simulink model "Demo002ADAS"  (Simulink 8.3)
settings: Solver=ode45  StartTime=0.0  StopTime=10.0  RelTol=1e-3
model workspace (MAT data in the model file):
  MPS_Models = {'..\..\..\solutions\demos\models\demos\Demo002.mps'}
  variantInfo = VariabilitySupport
  variantInfo.name = 'ADASVariabilityModel'
  variantInfo.configModels = VariantConfigurationModel
  variantInfo.configModels.id = '4psHK0ldtYh'
  variantInfo.configModels.name = 'PL_OEM1_AB01'
  variantInfo.configModels.featureRef = MpsObjectRef
  variantInfo.configModels.featureRef.targetNodeId = '4psHK0ldtYc'
  variantInfo.configModels.featureRef.resolveInfo = 'ADASVariabilityMdl'
  variantInfo.configModels.rootFeature = VariantSelectedFeature
  variantInfo.configModels.rootFeature.featureRef = MpsObjectRef
  variantInfo.configModels.rootFeature.featureRef.targetNodeId = '4psHK0ldtYd'
  variantInfo.configModels.rootFeature.featureRef.resolveInfo = 'ADASVariabilityMdl_root'
  variantInfo.configModels.rootFeature.children(1) = VariantSelectedFeature
  variantInfo.configModels.rootFeature.children(1).featureRef = MpsObjectRef
  variantInfo.configModels.rootFeature.children(1).featureRef.targetNodeId = '2wirY2bY5pP'
  variantInfo.configModels.rootFeature.children(1).featureRef.resolveInfo = 'ProductLine'
  variantInfo.configModels.rootFeature.children(1).children(1) = VariantSelectedFeature
  variantInfo.configModels.rootFeature.children(1).children(1).featureRef = MpsObjectRef
  variantInfo.configModels.rootFeature.children(1).children(1).featureRef.targetNodeId = '63tTPuP4CV9'
  variantInfo.configModels.rootFeature.children(1).children(1).featureRef.resolveInfo = 'Sensors'
  variantInfo.configModels.rootFeature.children(1).children(1).children = VariantSelectedFeature
  variantInfo.configModels.rootFeature.children(1).children(1).children.featureRef = MpsObjectRef
  variantInfo.configModels.rootFeature.children(1).children(1).children.featureRef.targetNodeId = '6jJ$2DnCoYq'
  variantInfo.configModels.rootFeature.children(1).children(1).children.featureRef.resolveInfo = 'Camera'
  variantInfo.configModels.rootFeature.children(1).children(1).children.children = VariantSelectedFeature
  variantInfo.configModels.rootFeature.children(1).children(1).children.children.featureRef = MpsObjectRef
  variantInfo.configModels.rootFeature.children(1).children(1).children.children.featureRef.targetNodeId = '6jJ$2DnCptI'
  variantInfo.configModels.rootFeature.children(1).children(1).children.children.featureRef.resolveInfo = 'C1'
  variantInfo.configModels.rootFeature.children(1).children(2) = VariantSelectedFeature
  variantInfo.configModels.rootFeature.children(1).children(2).featureRef = MpsObjectRef
  variantInfo.configModels.rootFeature.children(1).children(2).featureRef.targetNodeId = '6jJ$2DnCqGP'
  variantInfo.configModels.rootFeature.children(1).children(2).featureRef.resolveInfo = 'Actuators'
  variantInfo.configModels.rootFeature.children(1).children(2).children(1) = VariantSelectedFeature
  variantInfo.configModels.rootFeature.children(1).children(2).children(1).featureRef = MpsObjectRef
  variantInfo.configModels.rootFeature.children(1).children(2).children(1).featureRef.targetNodeId = '6jJ$2DnCqHv'
  variantInfo.configModels.rootFeature.children(1).children(2).children(1).featureRef.resolveInfo = 'PT'
  variantInfo.configModels.rootFeature.children(1).children(2).children(1).children = VariantSelectedFeature
  variantInfo.configModels.rootFeature.children(1).children(2).children(1).children.featureRef = MpsObjectRef
  variantInfo.configModels.rootFeature.children(1).children(2).children(1).children.featureRef.targetNodeId = '6jJ$2DnCqIu'
  variantInfo.configModels.rootFeature.children(1).children(2).children(1).children.featureRef.resolveInfo = 'G1'
  variantInfo.configModels.rootFeature.children(1).children(2).children(2) = VariantSelectedFeature
  variantInfo.configModels.rootFeature.children(1).children(2).children(2).featureRef = MpsObjectRef
  variantInfo.configModels.rootFeature.children(1).children(2).children(2).featureRef.targetNodeId = '6jJ$2DnCqHy'
  variantInfo.configModels.rootFeature.children(1).children(2).children(2).featureRef.resolveInfo = 'Brakes'
  variantInfo.configModels.rootFeature.children(1).children(2).children(2).children = VariantSelectedFeature
  variantInfo.configModels.rootFeature.children(1).children(2).children(2).children.featureRef = MpsObjectRef
  variantInfo.configModels.rootFeature.children(1).children(2).children(2).children.featureRef.targetNodeId = '6jJ$2DnCqYd'
  variantInfo.configModels.rootFeature.children(1).children(2).children(2).children.featureRef.resolveInfo = 'H1'
  variantInfo.configModels.rootFeature.children(1).children(2).children(3) = VariantSelectedFeature
  variantInfo.configModels.rootFeature.children(1).children(2).children(3).featureRef = MpsObjectRef
  variantInfo.configModels.rootFeature.children(1).children(2).children(3).featureRef.targetNodeId = '6jJ$2DnCqH_'
  variantInfo.configModels.rootFeature.children(1).children(2).children(3).featureRef.resolveInfo = 'Steering'
  variantInfo.configModels.rootFeature.children(1).children(2).children(3).children = VariantSelectedFeature
  variantInfo.configModels.rootFeature.children(1).children(2).children(3).children.featureRef = MpsObjectRef
  variantInfo.configModels.rootFeature.children(1).children(2).children(3).children.featureRef.targetNodeId = '6jJ$2DnCrdZ'
  variantInfo.configModels.rootFeature.children(1).children(2).children(3).children.featureRef.resolveInfo = 'I1'
  variantInfo.configModels.rootFeature.children(1).children(2).children(4) = VariantSelectedFeature
  variantInfo.configModels.rootFeature.children(1).children(2).children(4).featureRef = MpsObjectRef
  variantInfo.configModels.rootFeature.children(1).children(2).children(4).featureRef.targetNodeId = '6jJ$2DnCqHD'
  variantInfo.configModels.rootFeature.children(1).children(2).children(4).featureRef.resolveInfo = 'Headlight'
  variantInfo.configModels.rootFeature.children(1).children(2).children(4).children = VariantSelectedFeature
  variantInfo.configModels.rootFeature.children(1).children(2).children(4).children.featureRef = MpsObjectRef
  variantInfo.configModels.rootFeature.children(1).children(2).children(4).children.featureRef.targetNodeId = '6jJ$2DnCJBB'
  variantInfo.configModels.rootFeature.children(1).children(2).children(4).children.featureRef.resolveInfo = 'ToHLComm'
  variantInfo.configModels.rootFeature.children(1).children(2).children(5) = VariantSelectedFeature
  variantInfo.configModels.rootFeature.children(1).children(2).children(5).featureRef = MpsObjectRef
  variantInfo.configModels.rootFeature.children(1).children(2).children(5).featureRef.targetNodeId = '6jJ$2DnCqHI'
  variantInfo.configModels.rootFeature.children(1).children(2).children(5).featureRef.resolveInfo = 'IP'
  variantInfo.configModels.rootFeature.children(1).children(2).children(5).children = VariantSelectedFeature
  variantInfo.configModels.rootFeature.children(1).children(2).children(5).children.featureRef = MpsObjectRef
  variantInfo.configModels.rootFeature.children(1).children(2).children(5).children.featureRef.targetNodeId = '6jJ$2DnCrHG'
  variantInfo.configModels.rootFeature.children(1).children(2).children(5).children.featureRef.resolveInfo = 'K1'
  variantInfo.configModels.rootFeature.children(1).children(3) = VariantSelectedFeature
  variantInfo.configModels.rootFeature.children(1).children(3).featureRef = MpsObjectRef
  variantInfo.configModels.rootFeature.children(1).children(3).featureRef.targetNodeId = '63tTPuP4CVo'
  variantInfo.configModels.rootFeature.children(1).children(3).featureRef.resolveInfo = 'region'
  variantInfo.configModels.rootFeature.children(1).children(3).children = VariantSelectedFeature
  variantInfo.configModels.rootFeature.children(1).children(3).children.featureRef = MpsObjectRef
  variantInfo.configModels.rootFeature.children(1).children(3).children.featureRef.targetNodeId = '63tTPuP4CVv'
  variantInfo.configModels.rootFeature.children(1).children(3).children.featureRef.resolveInfo = 'Germany'
  variantInfo.configModels.rootFeature.children(1).children(4) = VariantSelectedFeature
  variantInfo.configModels.rootFeature.children(1).children(4).featureRef = MpsObjectRef
  variantInfo.configModels.rootFeature.children(1).children(4).featureRef.targetNodeId = '6jJ$2DnCrX_'
  variantInfo.configModels.rootFeature.children(1).children(4).featureRef.resolveInfo = 'MajorFunctions'
  variantInfo.configModels.rootFeature.children(1).children(4).children = VariantSelectedFeature
  variantInfo.configModels.rootFeature.children(1).children(4).children.featureRef = MpsObjectRef
  variantInfo.configModels.rootFeature.children(1).children(4).children.featureRef.targetNodeId = '6jJ$2DnCrYD'
  variantInfo.configModels.rootFeature.children(1).children(4).children.featureRef.resolveInfo = 'TSR'
  variantInfo.configModels.rootFeature.children(1).children(5) = VariantSelectedFeature
  variantInfo.configModels.rootFeature.children(1).children(5).featureRef = MpsObjectRef
  variantInfo.configModels.rootFeature.children(1).children(5).featureRef.targetNodeId = '6jJ$2DnCJfc'
  variantInfo.configModels.rootFeature.children(1).children(5).featureRef.resolveInfo = 'Customer'
  variantInfo.configModels.rootFeature.children(1).children(6) = VariantSelectedFeature
  variantInfo.configModels.rootFeature.children(1).children(6).featureRef = MpsObjectRef
  variantInfo.configModels.rootFeature.children(1).children(6).featureRef.targetNodeId = '6jJ$2DnCJd5'
  variantInfo.configModels.rootFeature.children(1).children(6).featureRef.resolveInfo = 'Comm'
  variantInfo.configModels.rootFeature.children(2) = VariantSelectedFeature
  variantInfo.configModels.rootFeature.children(2).featureRef = MpsObjectRef
  variantInfo.configModels.rootFeature.children(2).featureRef.targetNodeId = '2wirY2bYc6v'
  variantInfo.configModels.rootFeature.children(2).featureRef.resolveInfo = 'ProductTesting'
  variantInfo.configModels.rootFeature.children(2).children = VariantSelectedFeature
  variantInfo.configModels.rootFeature.children(2).children.featureRef = MpsObjectRef
  variantInfo.configModels.rootFeature.children(2).children.featureRef.targetNodeId = '2wirY2bYc8b'
  variantInfo.configModels.rootFeature.children(2).children.featureRef.resolveInfo = 'MIL'
PreLoadFcn:
  | VarScript002ADAS
PostLoadFcn:
  | loadDRIReqsInfo('Demo002ADAS', []);
PreSaveFcn:
  | modelWS=get_param('Demo002ADAS', 'modelworkspace');modelWS.evalin('clear driModuleInfo simModuleInfo');clear modelWS;
settings Model: Creator=swami  LastModifiedBy=swami
settings DataIOCC: SignalLoggingSaveFormat=Dataset
settings DebuggingCC: UnderspecifiedInitializationDetection=Simplified  StateNameClashWarn=none
settings GRTTargetCC: CombineOutputUpdateFcns=on  GRTInterface=off

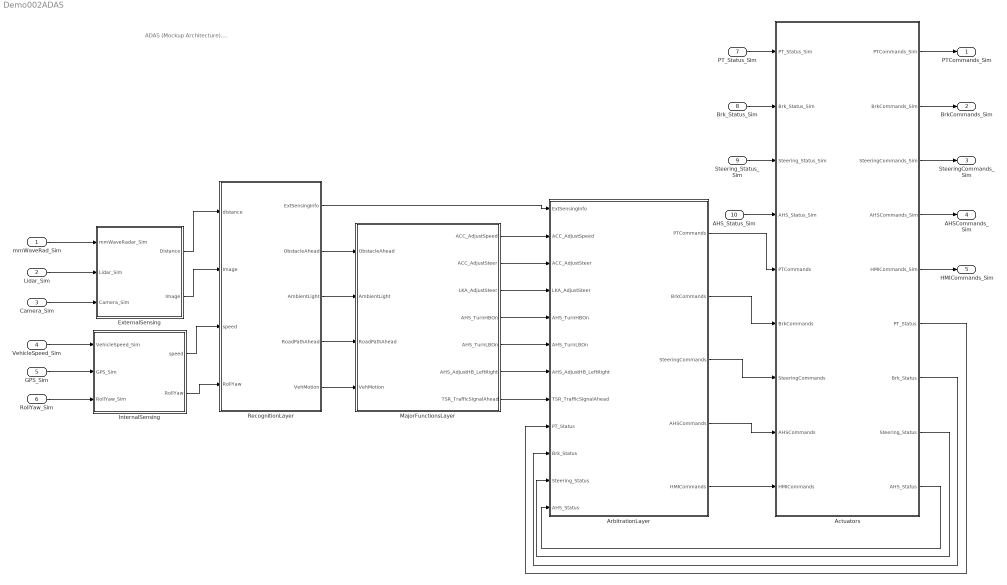
== system Demo002ADAS ==
  note: ADAS (Mockup Architecture)....
  mmWaveRad_Sim : Inport
  Lidar_Sim : Inport  Port=2
  Camera_Sim : Inport  Port=3
  VehicleSpeed_Sim : Inport  Port=4
  GPS_Sim : Inport  Port=5
  RollYaw_Sim : Inport  Port=6
  PT_Status_Sim : Inport  Port=7
  Brk_Status_Sim : Inport  Port=8
  Steering_Status_Sim : Inport  Port=9
  AHS_Status_Sim : Inport  Port=10
  Actuators : Subsystem
  ArbitrationLayer : Subsystem
  ExternalSensing : Subsystem
  InternalSensing : Subsystem
  MajorFunctionsLayer : Subsystem
  RecognitionLayer : Subsystem
  PTCommands_Sim : Outport
  BrkCommands_Sim : Outport  Port=2
  SteeringCommands_Sim : Outport  Port=3
  AHSCommands_Sim : Outport  Port=4
  HMICommands_Sim : Outport  Port=5
  wires:
  MajorFunctionsLayer/1(ACC_AdjustSpeed) -> ArbitrationLayer/2(ACC_AdjustSpeed)
  MajorFunctionsLayer/2(ACC_AdjustSteer) -> ArbitrationLayer/3(ACC_AdjustSteer)
  MajorFunctionsLayer/3(LKA_AdjustSteer) -> ArbitrationLayer/4(LKA_AdjustSteer)
  MajorFunctionsLayer/4(AHS_TurnHBOn) -> ArbitrationLayer/5(AHS_TurnHBOn)
  MajorFunctionsLayer/5(AHS_TurnLBOn) -> ArbitrationLayer/6(AHS_TurnLBOn)
  MajorFunctionsLayer/6(AHS_AdjustHB_LeftRight) -> ArbitrationLayer/7(AHS_AdjustHB_LeftRight)
  MajorFunctionsLayer/7(TSR_TrafficSignalAhead) -> ArbitrationLayer/8(TSR_TrafficSIgnalAhead)
  RecognitionLayer/2(ObstacleAhead) -> MajorFunctionsLayer/1(ObstacleAhead)
  RecognitionLayer/3(AmbientLight) -> MajorFunctionsLayer/2(AmbientLight)
  RecognitionLayer/4(RoadPathAhead) -> MajorFunctionsLayer/3(RoadPathAhead)
  RecognitionLayer/5(VehMotion) -> MajorFunctionsLayer/4(VehMotion)
  ExternalSensing/2(Image) -> RecognitionLayer/2(Image)
  ExternalSensing/1(Distance) -> RecognitionLayer/1(distance)
  InternalSensing/1(speed) -> RecognitionLayer/3(speed)
  InternalSensing/2(RollYaw) -> RecognitionLayer/4(RollYaw)
  ArbitrationLayer/2(BrkCommands) -> Actuators/6(BrkCommands)
  ArbitrationLayer/4(AHSCommands) -> Actuators/8(AHSCommands)
  ArbitrationLayer/5(HMICommands) -> Actuators/9(HMICommands)
  Actuators/9(AHS_Status) -> ArbitrationLayer/12(AHS_Status)
  RecognitionLayer/1(ExtSensingInfo) -> ArbitrationLayer/1(ExtSensingInfo)
  Actuators/1(PTCommands_Sim) -> PTCommands_Sim/1
  Actuators/2(BrkCommands_Sim) -> BrkCommands_Sim/1
  Actuators/3(SteeringCommands_Sim) -> SteeringCommands_Sim/1
  Actuators/4(AHSCommands_Sim) -> AHSCommands_Sim/1
  Actuators/5(HMICommands_Sim) -> HMICommands_Sim/1
  mmWaveRad_Sim/1 -> ExternalSensing/1(mmWaveRadar_Sim)
  Lidar_Sim/1 -> ExternalSensing/2(Lidar_Sim)
  Camera_Sim/1 -> ExternalSensing/3(Camera_Sim)
  VehicleSpeed_Sim/1 -> InternalSensing/1(VehicleSpeed_Sim)
  RollYaw_Sim/1 -> InternalSensing/3(RollYaw_Sim)
  GPS_Sim/1 -> InternalSensing/2(GPS_Sim)
  Actuators/8(Steering_Status) -> ArbitrationLayer/11(Steering_Status)
  Actuators/7(Brk_Status) -> ArbitrationLayer/10(Brk_Status)
  Actuators/6(PT_Status) -> ArbitrationLayer/9(PT_Status)
  PT_Status_Sim/1 -> Actuators/1(PT_Status_Sim)
  Brk_Status_Sim/1 -> Actuators/2(Brk_Status_Sim)
  Steering_Status_Sim/1 -> Actuators/3(Steering_Status_Sim)
  AHS_Status_Sim/1 -> Actuators/4(AHS_Status_Sim)
  ArbitrationLayer/1(PTCommands) -> Actuators/5(PTCommands)
  ArbitrationLayer/3(SteeringCommands) -> Actuators/7(SteeringCommands)

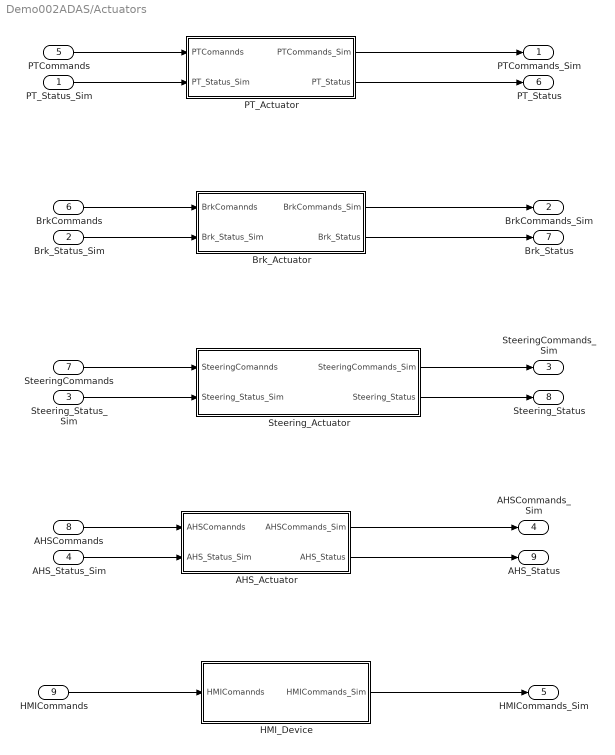
== system Demo002ADAS/Actuators ==
  PT_Status_Sim : Inport
  Brk_Status_Sim : Inport  Port=2
  Steering_Status_Sim : Inport  Port=3
  AHS_Status_Sim : Inport  Port=4
  PTCommands : Inport  Port=5
  BrkCommands : Inport  Port=6
  SteeringCommands : Inport  Port=7
  AHSCommands : Inport  Port=8
  HMICommands : Inport  Port=9
  AHS_Actuator : Subsystem  Variant=on
  Brk_Actuator : Subsystem  Variant=on
  HMI_Device : Subsystem  Variant=on
  PT_Actuator : Subsystem  Variant=on
  Steering_Actuator : Subsystem  Variant=on
  PTCommands_Sim : Outport
  BrkCommands_Sim : Outport  Port=2
  SteeringCommands_Sim : Outport  Port=3
  AHSCommands_Sim : Outport  Port=4
  HMICommands_Sim : Outport  Port=5
  PT_Status : Outport  Port=6
  Brk_Status : Outport  Port=7
  Steering_Status : Outport  Port=8
  AHS_Status : Outport  Port=9
  wires:
  PTCommands/1 -> PT_Actuator/1(PTComannds)
  PT_Actuator/1(PTCommands_Sim) -> PTCommands_Sim/1
  PT_Actuator/2(PT_Status) -> PT_Status/1
  BrkCommands/1 -> Brk_Actuator/1(BrkComannds)
  Brk_Actuator/1(BrkCommands_Sim) -> BrkCommands_Sim/1
  Brk_Actuator/2(Brk_Status) -> Brk_Status/1
  SteeringCommands/1 -> Steering_Actuator/1(SteeringComannds)
  Steering_Actuator/1(SteeringCommands_Sim) -> SteeringCommands_Sim/1
  Steering_Actuator/2(Steering_Status) -> Steering_Status/1
  AHSCommands/1 -> AHS_Actuator/1(AHSComannds)
  AHS_Actuator/1(AHSCommands_Sim) -> AHSCommands_Sim/1
  AHS_Actuator/2(AHS_Status) -> AHS_Status/1
  HMICommands/1 -> HMI_Device/1(HMIComannds)
  HMI_Device/1(HMICommands_Sim) -> HMICommands_Sim/1
  PT_Status_Sim/1 -> PT_Actuator/2(PT_Status_Sim)
  Brk_Status_Sim/1 -> Brk_Actuator/2(Brk_Status_Sim)
  Steering_Status_Sim/1 -> Steering_Actuator/2(Steering_Status_Sim)
  AHS_Status_Sim/1 -> AHS_Actuator/2(AHS_Status_Sim)

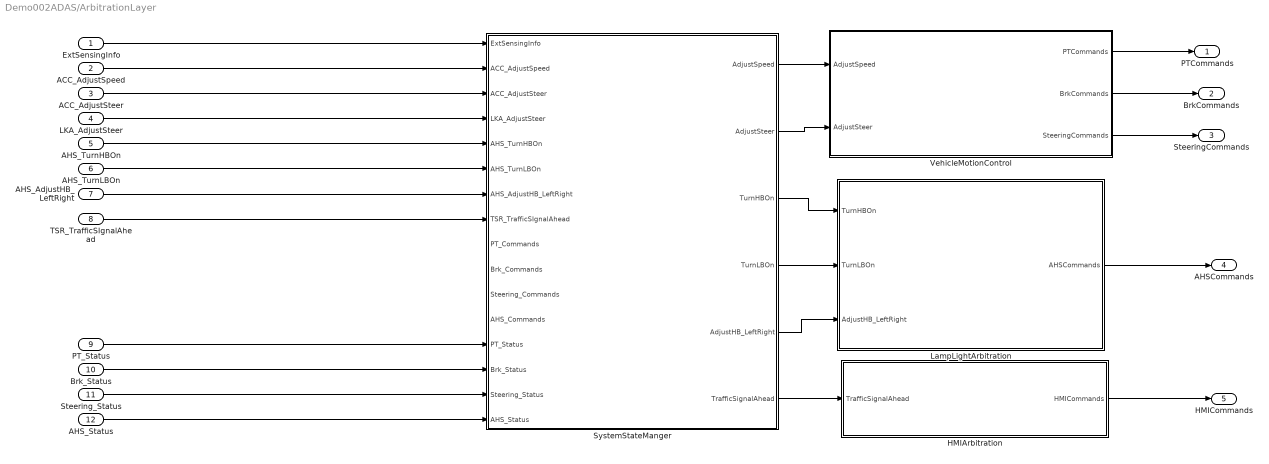
== system Demo002ADAS/ArbitrationLayer ==
  ExtSensingInfo : Inport
  ACC_AdjustSpeed : Inport  Port=2
  ACC_AdjustSteer : Inport  Port=3
  LKA_AdjustSteer : Inport  Port=4
  AHS_TurnHBOn : Inport  Port=5
  AHS_TurnLBOn : Inport  Port=6
  AHS_AdjustHB_LeftRight : Inport  Port=7
  TSR_TrafficSIgnalAhead : Inport  Port=8
  PT_Status : Inport  Port=9
  Brk_Status : Inport  Port=10
  Steering_Status : Inport  Port=11
  AHS_Status : Inport  Port=12
  HMIArbitration : Subsystem  Variant=on
  LampLightArbitration : Subsystem  Variant=on
  SystemStateManger : Subsystem  Variant=on
  VehicleMotionControl : Subsystem
  PTCommands : Outport
  BrkCommands : Outport  Port=2
  SteeringCommands : Outport  Port=3
  AHSCommands : Outport  Port=4
  HMICommands : Outport  Port=5
  wires:
  ACC_AdjustSpeed/1 -> SystemStateManger/2(ACC_AdjustSpeed)
  ACC_AdjustSteer/1 -> SystemStateManger/3(ACC_AdjustSteer)
  LKA_AdjustSteer/1 -> SystemStateManger/4(LKA_AdjustSteer)
  AHS_TurnHBOn/1 -> SystemStateManger/5(AHS_TurnHBOn)
  AHS_TurnLBOn/1 -> SystemStateManger/6(AHS_TurnLBOn)
  AHS_AdjustHB_LeftRight/1 -> SystemStateManger/7(AHS_AdjustHB_LeftRight)
  TSR_TrafficSIgnalAhead/1 -> SystemStateManger/8(TSR_TrafficSIgnalAhead)
  PT_Status/1 -> SystemStateManger/13(PT_Status)
  Brk_Status/1 -> SystemStateManger/14(Brk_Status)
  Steering_Status/1 -> SystemStateManger/15(Steering_Status)
  AHS_Status/1 -> SystemStateManger/16(AHS_Status)
  SystemStateManger/1(AdjustSpeed) -> VehicleMotionControl/1(AdjustSpeed)
  SystemStateManger/2(AdjustSteer) -> VehicleMotionControl/2(AdjustSteer)
  VehicleMotionControl/1(PTCommands) -> PTCommands/1
  VehicleMotionControl/2(BrkCommands) -> BrkCommands/1
  VehicleMotionControl/3(SteeringCommands) -> SteeringCommands/1
  SystemStateManger/3(TurnHBOn) -> LampLightArbitration/1(TurnHBOn)
  SystemStateManger/4(TurnLBOn) -> LampLightArbitration/2(TurnLBOn)
  SystemStateManger/5(AdjustHB_LeftRight) -> LampLightArbitration/3(AdjustHB_LeftRight)
  LampLightArbitration/1(AHSCommands) -> AHSCommands/1
  SystemStateManger/6(TrafficSignalAhead) -> HMIArbitration/1(TrafficSignalAhead)
  HMIArbitration/1(HMICommands) -> HMICommands/1
  ExtSensingInfo/1 -> SystemStateManger/1(ExtSensingInfo)

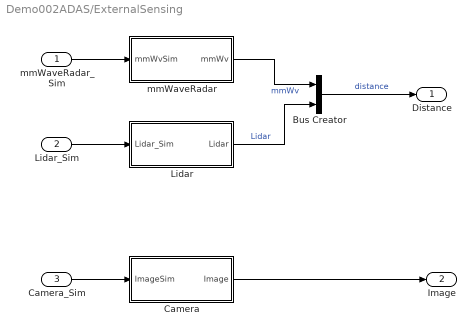
== system Demo002ADAS/ExternalSensing ==
  mmWaveRadar_Sim : Inport
  Lidar_Sim : Inport  Port=2
  Camera_Sim : Inport  Port=3
  Bus Creator : BusCreator  Inputs=2
  Camera : Subsystem  Variant=on
  Lidar : Subsystem  Variant=on
  mmWaveRadar : Subsystem  Variant=on
  Distance : Outport
  Image : Outport  Port=2
  wires:
  mmWaveRadar_Sim/1 -> mmWaveRadar/1(mmWvSim)
  mmWaveRadar/1(mmWv) -> Bus Creator/1  "mmWv"
  Lidar_Sim/1 -> Lidar/1(Lidar_Sim)
  Lidar/1(Lidar) -> Bus Creator/2  "Lidar"
  Bus Creator/1 -> Distance/1  "distance"
  Camera/1(Image) -> Image/1
  Camera_Sim/1 -> Camera/1(ImageSim)

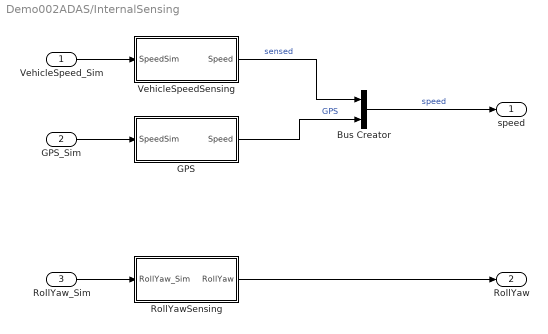
== system Demo002ADAS/InternalSensing ==
  VehicleSpeed_Sim : Inport
  GPS_Sim : Inport  Port=2
  RollYaw_Sim : Inport  Port=3
  Bus Creator : BusCreator  Inputs=2
  GPS : Subsystem  Variant=on
  RollYawSensing : Subsystem  Variant=on
  VehicleSpeedSensing : Subsystem  Variant=on
  speed : Outport
  RollYaw : Outport  Port=2
  wires:
  RollYaw_Sim/1 -> RollYawSensing/1(RollYaw_Sim)
  RollYawSensing/1(RollYaw) -> RollYaw/1
  VehicleSpeed_Sim/1 -> VehicleSpeedSensing/1(SpeedSim)
  GPS_Sim/1 -> GPS/1(SpeedSim)
  VehicleSpeedSensing/1(Speed) -> Bus Creator/1  "sensed"
  GPS/1(Speed) -> Bus Creator/2  "GPS"
  Bus Creator/1 -> speed/1  "speed"

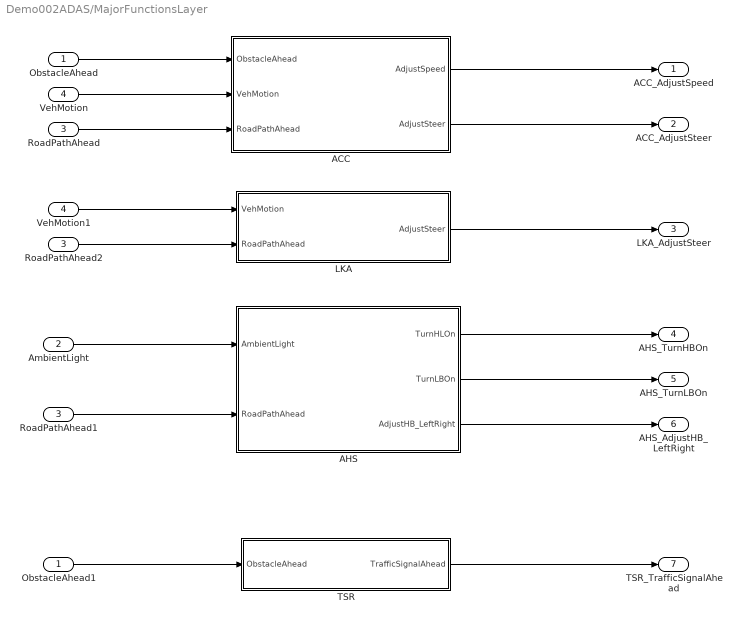
== system Demo002ADAS/MajorFunctionsLayer ==
  ObstacleAhead : Inport
  AmbientLight : Inport  Port=2
  RoadPathAhead : Inport  Port=3
  VehMotion : Inport  Port=4
  ACC : Subsystem  Variant=on
  AHS : Subsystem  Variant=on
  LKA : Subsystem  Variant=on
  ObstacleAhead1 : InportShadow
  RoadPathAhead1 : InportShadow  Port=3
  RoadPathAhead2 : InportShadow  Port=3
  TSR : Subsystem  Variant=on
  VehMotion1 : InportShadow  Port=4
  ACC_AdjustSpeed : Outport
  ACC_AdjustSteer : Outport  Port=2
  LKA_AdjustSteer : Outport  Port=3
  AHS_TurnHBOn : Outport  Port=4
  AHS_TurnLBOn : Outport  Port=5
  AHS_AdjustHB_LeftRight : Outport  Port=6
  TSR_TrafficSignalAhead : Outport  Port=7
  wires:
  LKA/1(AdjustSteer) -> LKA_AdjustSteer/1
  AmbientLight/1 -> AHS/1(AmbientLight)
  TSR/1(TrafficSignalAhead) -> TSR_TrafficSignalAhead/1
  ObstacleAhead/1 -> ACC/1(ObstacleAhead)
  ACC/1(AdjustSpeed) -> ACC_AdjustSpeed/1
  VehMotion1/1 -> LKA/1(VehMotion)
  ObstacleAhead1/1 -> TSR/1(ObstacleAhead)
  ACC/2(AdjustSteer) -> ACC_AdjustSteer/1
  VehMotion/1 -> ACC/2(VehMotion)
  RoadPathAhead/1 -> ACC/3(RoadPathAhead)
  AHS/1(TurnHLOn) -> AHS_TurnHBOn/1
  AHS/2(TurnLBOn) -> AHS_TurnLBOn/1
  AHS/3(AdjustHB_LeftRight) -> AHS_AdjustHB_LeftRight/1
  RoadPathAhead1/1 -> AHS/2(RoadPathAhead)
  RoadPathAhead2/1 -> LKA/2(RoadPathAhead)

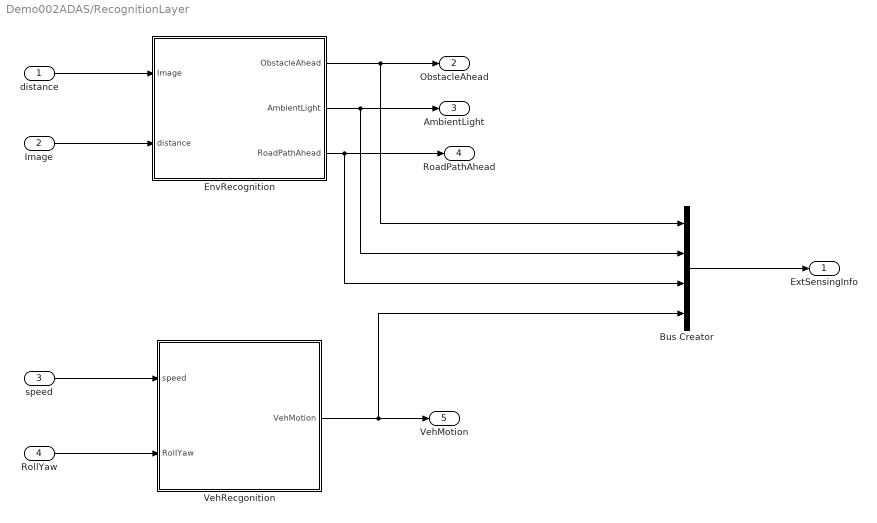
== system Demo002ADAS/RecognitionLayer ==
  distance : Inport
  Image : Inport  Port=2
  speed : Inport  Port=3
  RollYaw : Inport  Port=4
  Bus Creator : BusCreator
  EnvRecognition : Subsystem
  VehRecgonition : Subsystem
  ExtSensingInfo : Outport
  ObstacleAhead : Outport  Port=2
  AmbientLight : Outport  Port=3
  RoadPathAhead : Outport  Port=4
  VehMotion : Outport  Port=5
  wires:
  distance/1 -> EnvRecognition/1(Image)
  Image/1 -> EnvRecognition/2(distance)
  EnvRecognition/1(ObstacleAhead) -> Bus Creator/1, ObstacleAhead/1
  EnvRecognition/2(AmbientLight) -> Bus Creator/2, AmbientLight/1
  speed/1 -> VehRecgonition/1(speed)
  RollYaw/1 -> VehRecgonition/2(RollYaw)
  EnvRecognition/3(RoadPathAhead) -> Bus Creator/3, RoadPathAhead/1
  Bus Creator/1 -> ExtSensingInfo/1
  VehRecgonition/1(VehMotion) -> Bus Creator/4, VehMotion/1

== system Demo002ADAS/Actuators/AHS_Actuator ==
  note: 1) Only subsystems can be added as variant choices at this level
      | 2) Blocks cannot be connected at this level as connectivity is
      | automatically determined at simulation, based on the active variant
  AHSComannds : Inport
  AHS_Status_Sim : Inport  Port=2
  Actuator_J1 : Subsystem  VariantControl=D2_Act_AHS_Actuator_Actuator_J1
  Actuator_J2 : Subsystem  VariantControl=D2_Act_AHS_Actuator_Actuator_J2
  ToHIL : Subsystem  VariantControl=D2_Act_AHS_Actuator_ToHIL
  ToSimulation : Subsystem  VariantControl=D2_Act_AHS_Actuator_ToSimulation
  AHSCommands_Sim : Outport
  AHS_Status : Outport  Port=2

== system Demo002ADAS/Actuators/Brk_Actuator ==
  note: 1) Only subsystems can be added as variant choices at this level
      | 2) Blocks cannot be connected at this level as connectivity is
      | automatically determined at simulation, based on the active variant
  BrkComannds : Inport
  Brk_Status_Sim : Inport  Port=2
  Actuator_H1 : Subsystem  VariantControl=D2_Act_Brk_Actuator_Actuator_H1
  Actuator_H2 : Subsystem  VariantControl=D2_Act_Brk_Actuator_Actuator_H2
  ToHIL : Subsystem  VariantControl=D2_Act_Brk_Actuator_ToHIL
  ToSimulation : Subsystem  VariantControl=D2_Act_Brk_Actuator_ToSimulation
  BrkCommands_Sim : Outport
  Brk_Status : Outport  Port=2

== system Demo002ADAS/Actuators/HMI_Device ==
  note: 1) Only subsystems can be added as variant choices at this level
      | 2) Blocks cannot be connected at this level as connectivity is
      | automatically determined at simulation, based on the active variant
  HMIComannds : Inport
  IP_K1 : Subsystem  VariantControl=D2_Act_HMI_Device_IP_K1
  IP_K2 : Subsystem  VariantControl=D2_Act_HMI_Device_IP_K2
  ToHIL : Subsystem  VariantControl=D2_Act_HMI_Device_ToHIL
  ToSimulation : Subsystem  VariantControl=D2_Act_HMI_Device_ToSimulation
  HMICommands_Sim : Outport

== system Demo002ADAS/Actuators/PT_Actuator ==
  note: 1) Only subsystems can be added as variant choices at this level
      | 2) Blocks cannot be connected at this level as connectivity is
      | automatically determined at simulation, based on the active variant
  PTComannds : Inport
  PT_Status_Sim : Inport  Port=2
  Actuator_G1 : Subsystem  VariantControl=D2_Act_PT_Actuator_Actuator_G1
  Actuator_G2 : Subsystem  VariantControl=D2_Act_PT_Actuator_Actuator_G2
  ToHIL : Subsystem  VariantControl=D2_Act_PT_Actuator_ToHIL
  ToSimulation : Subsystem  VariantControl=D2_Act_PT_Actuator_ToSimulation
  PTCommands_Sim : Outport
  PT_Status : Outport  Port=2

== system Demo002ADAS/Actuators/Steering_Actuator ==
  note: 1) Only subsystems can be added as variant choices at this level
      | 2) Blocks cannot be connected at this level as connectivity is
      | automatically determined at simulation, based on the active variant
  SteeringComannds : Inport
  Steering_Status_Sim : Inport  Port=2
  Actuator_I1 : Subsystem  VariantControl=D2_Act_Steering_Actuator_Actuator_I1
  ToHIL : Subsystem  VariantControl=D2_Act_Steering_Actuator_ToHIL
  ToSimulation : Subsystem  VariantControl=D2_Act_Steering_Actuator_ToSimulation
  SteeringCommands_Sim : Outport
  Steering_Status : Outport  Port=2

== system Demo002ADAS/ArbitrationLayer/HMIArbitration ==
  note: 1) Only subsystems can be added as variant choices at this level
      | 2) Blocks cannot be connected at this level as connectivity is
      | automatically determined at simulation, based on the active variant
  TrafficSignalAhead : Inport
  IP_K1 : Subsystem  VariantControl=D2_AL_HMIArbitration_IP_K1
  IP_K2 : Subsystem  VariantControl=D2_AL_HMIArbitration_IP_K2
  ToSimulationAndHIL : Subsystem  VariantControl=D2_AL_HMIArbitration_ToSimulationAndHIL
  HMICommands : Outport

== system Demo002ADAS/ArbitrationLayer/LampLightArbitration ==
  note: 1) Only subsystems can be added as variant choices at this level
      | 2) Blocks cannot be connected at this level as connectivity is
      | automatically determined at simulation, based on the active variant
  TurnHBOn : Inport
  TurnLBOn : Inport  Port=2
  AdjustHB_LeftRight : Inport  Port=3
  Actuator_J2 : Subsystem  VariantControl=D2_AL_LampLightArbitration_Actuator_J2
  "ToSimulation, HIL, and Actuator_J1" : Subsystem  VariantControl=D2_AL_LampLightArbitration_ToSimulation_HIL_and_Actuator_J1
  AHSCommands : Outport

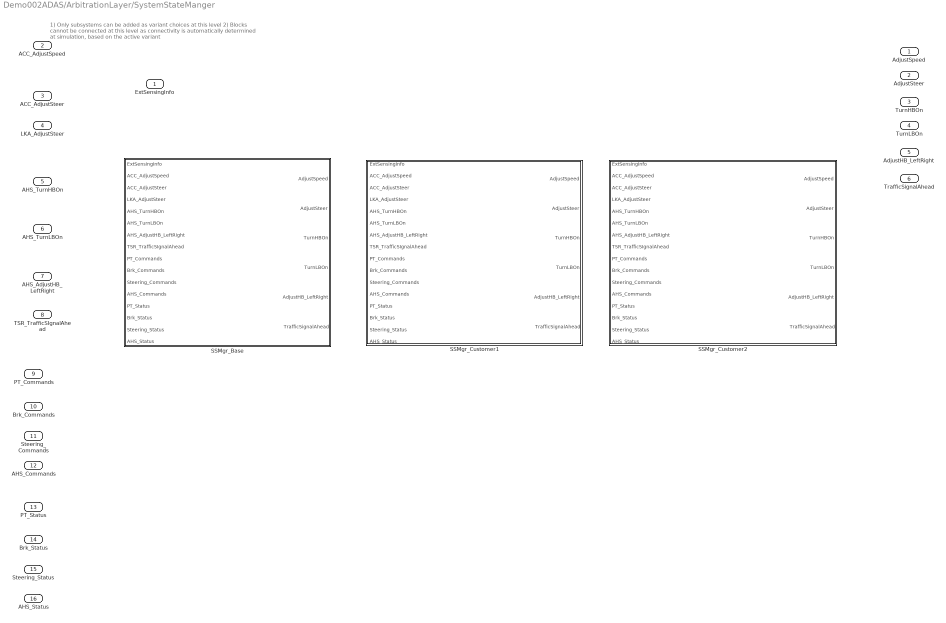
== system Demo002ADAS/ArbitrationLayer/SystemStateManger ==
  note: 1) Only subsystems can be added as variant choices at this level
      | 2) Blocks cannot be connected at this level as connectivity is
      | automatically determined at simulation, based on the active variant
  ExtSensingInfo : Inport
  ACC_AdjustSpeed : Inport  Port=2
  ACC_AdjustSteer : Inport  Port=3
  LKA_AdjustSteer : Inport  Port=4
  AHS_TurnHBOn : Inport  Port=5
  AHS_TurnLBOn : Inport  Port=6
  AHS_AdjustHB_LeftRight : Inport  Port=7
  TSR_TrafficSIgnalAhead : Inport  Port=8
  PT_Commands : Inport  Port=9
  Brk_Commands : Inport  Port=10
  Steering_Commands : Inport  Port=11
  AHS_Commands : Inport  Port=12
  PT_Status : Inport  Port=13
  Brk_Status : Inport  Port=14
  Steering_Status : Inport  Port=15
  AHS_Status : Inport  Port=16
  SSMgr_Base : Subsystem  VariantControl=D2_AL_SystemStateManger_SSMgr_Base
  SSMgr_Customer1 : Subsystem  VariantControl=D2_AL_SystemStateManger_SSMgr_Customer1
  SSMgr_Customer2 : Subsystem  VariantControl=D2_AL_SystemStateManger_SSMgr_Customer2
  AdjustSpeed : Outport
  AdjustSteer : Outport  Port=2
  TurnHBOn : Outport  Port=3
  TurnLBOn : Outport  Port=4
  AdjustHB_LeftRight : Outport  Port=5
  TrafficSignalAhead : Outport  Port=6

== system Demo002ADAS/ArbitrationLayer/VehicleMotionControl ==
  AdjustSpeed : Inport
  AdjustSteer : Inport  Port=2
  ForeAftMotion : Subsystem  Variant=on
  LeftRightMotion : Subsystem  Variant=on
  PTCommands : Outport
  BrkCommands : Outport  Port=2
  SteeringCommands : Outport  Port=3
  wires:
  AdjustSteer/1 -> LeftRightMotion/1(AdjustSteer)
  LeftRightMotion/1(SteeringCommands) -> SteeringCommands/1
  AdjustSpeed/1 -> ForeAftMotion/1(AdjustSpeed)
  ForeAftMotion/1(PTCommands) -> PTCommands/1
  ForeAftMotion/2(BrkCommands) -> BrkCommands/1

== system Demo002ADAS/ExternalSensing/Camera ==
  note: 1) Only subsystems can be added as variant choices at this level
      | 2) Blocks cannot be connected at this level as connectivity is
      | automatically determined at simulation, based on the active variant
  ImageSim : Inport
  FromHIL : Subsystem  VariantControl=D2_XSen_Camera_FromHIL
  FromSimulation : Subsystem  VariantControl=D2_XSen_Camera_FromSimulation
  Sensor_C1 : Subsystem  VariantControl=D2_XSen_Camera_Sensor_C1
  Sensor_C2 : Subsystem  VariantControl=D2_XSen_Camera_Sensor_C2
  Image : Outport

== system Demo002ADAS/ExternalSensing/Lidar ==
  note: 1) Only subsystems can be added as variant choices at this level
      | 2) Blocks cannot be connected at this level as connectivity is
      | automatically determined at simulation, based on the active variant
  Lidar_Sim : Inport
  FromHIL : Subsystem  VariantControl=D2_XSen_Lidar_FromHIL
  FromSimulation : Subsystem  VariantControl=D2_XSen_Lidar_FromSimulation
  Sensor_B1 : Subsystem  VariantControl=D2_XSen_Lidar_Sensor_B1
  Sensor_B2 : Subsystem  VariantControl=D2_XSen_Lidar_Sensor_B2
  Lidar : Outport

== system Demo002ADAS/ExternalSensing/mmWaveRadar ==
  note: 1) Only subsystems can be added as variant choices at this level
      | 2) Blocks cannot be connected at this level as connectivity is
      | automatically determined at simulation, based on the active variant
  mmWvSim : Inport
  FromHIL : Subsystem  VariantControl=D2_XSen_mmWaveRadar_FromHIL
  FromSimulation : Subsystem  VariantControl=D2_XSen_mmWaveRadar_FromSimulation
  Sensor_A1 : Subsystem  VariantControl=D2_XSen_mmWaveRadar_Sensor_A1
  Sensor_A2 : Subsystem  VariantControl=D2_XSen_mmWaveRadar_Sensor_A2
  mmWv : Outport

== system Demo002ADAS/InternalSensing/GPS ==
  note: 1) Only subsystems can be added as variant choices at this level
      | 2) Blocks cannot be connected at this level as connectivity is
      | automatically determined at simulation, based on the active variant
  SpeedSim : Inport
  FromHIL : Subsystem  VariantControl=D2_ISen_GPS_FromHIL
  FromSimulation : Subsystem  VariantControl=D2_ISen_GPS_FromSimulation
  GPS_E1 : Subsystem  VariantControl=D2_ISen_GPS_GPS_E1
  GPS_E2 : Subsystem  VariantControl=D2_ISen_GPS_GPS_E2
  Speed : Outport

== system Demo002ADAS/InternalSensing/RollYawSensing ==
  note: 1) Only subsystems can be added as variant choices at this level
      | 2) Blocks cannot be connected at this level as connectivity is
      | automatically determined at simulation, based on the active variant
  RollYaw_Sim : Inport
  FromHIL : Subsystem  VariantControl=D2_ISen_RollYawSensing_FromHIL
  FromSimulation : Subsystem  VariantControl=D2_ISen_RollYawSensing_FromSimulation
  Sensor_F1 : Subsystem  VariantControl=D2_ISen_RollYawSensing_Sensor_F1
  RollYaw : Outport

== system Demo002ADAS/InternalSensing/VehicleSpeedSensing ==
  note: 1) Only subsystems can be added as variant choices at this level
      | 2) Blocks cannot be connected at this level as connectivity is
      | automatically determined at simulation, based on the active variant
  SpeedSim : Inport
  FromComm : Subsystem  VariantControl=D2_ISen_VehicleSpeedSensing_FromComm
  FromHIL : Subsystem  VariantControl=D2_ISen_VehicleSpeedSensing_FromHIL
  FromSimulation : Subsystem  VariantControl=D2_ISen_VehicleSpeedSensing_FromSimulation
  Sensor_D1 : Subsystem  VariantControl=D2_ISen_VehicleSpeedSensing_Sensor_D1
  Sensor_D2 : Subsystem  VariantControl=D2_ISen_VehicleSpeedSensing_Sensor_D2
  Speed : Outport

== system Demo002ADAS/MajorFunctionsLayer/ACC ==
  note: 1) Only subsystems can be added as variant choices at this level
      | 2) Blocks cannot be connected at this level as connectivity is
      | automatically determined at simulation, based on the active variant
  ObstacleAhead : Inport
  VehMotion : Inport  Port=2
  RoadPathAhead : Inport  Port=3
  ACC_Complex : Subsystem  VariantControl=D2_MFL_ACC_ACC_Complex
  ACC_Simple : Subsystem  VariantControl=D2_MFL_ACC_ACC_Simple
  AdjustSpeed : Outport
  AdjustSteer : Outport  Port=2

== system Demo002ADAS/MajorFunctionsLayer/AHS ==
  note: 1) Only subsystems can be added as variant choices at this level
      | 2) Blocks cannot be connected at this level as connectivity is
      | automatically determined at simulation, based on the active variant
  AmbientLight : Inport
  RoadPathAhead : Inport  Port=2
  AHB_advanced : Subsystem  VariantControl=D2_MFL_AHS_AHB_advanced
  AHB_simple : Subsystem  VariantControl=D2_MFL_AHS_AHB_simple
  AHS : Subsystem  VariantControl=D2_MFL_AHS_AHS
  TurnHLOn : Outport
  TurnLBOn : Outport  Port=2
  AdjustHB_LeftRight : Outport  Port=3

== system Demo002ADAS/MajorFunctionsLayer/LKA ==
  note: 1) Only subsystems can be added as variant choices at this level
      | 2) Blocks cannot be connected at this level as connectivity is
      | automatically determined at simulation, based on the active variant
  VehMotion : Inport
  RoadPathAhead : Inport  Port=2
  LKA : Subsystem  VariantControl=D2_MFL_LKA_LKA
  AdjustSteer : Outport

== system Demo002ADAS/MajorFunctionsLayer/TSR ==
  note: 1) Only subsystems can be added as variant choices at this level
      | 2) Blocks cannot be connected at this level as connectivity is
      | automatically determined at simulation, based on the active variant
  ObstacleAhead : Inport
  TSR_Germany : Subsystem  VariantControl=D2_MFL_TSR_TSR_Germany
  TSR_Japan : Subsystem  VariantControl=D2_MFL_TSR_TSR_Japan
  TSR_UK : Subsystem  VariantControl=D2_MFL_TSR_TSR_UK
  TSR_US : Subsystem  VariantControl=D2_MFL_TSR_TSR_US
  TrafficSignalAhead : Outport

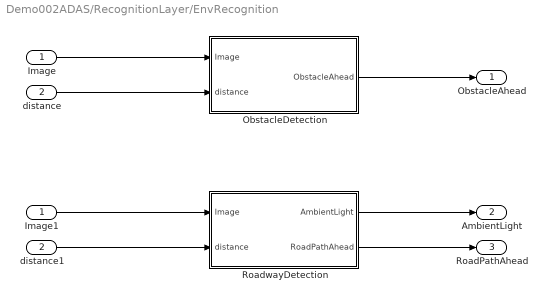
== system Demo002ADAS/RecognitionLayer/EnvRecognition ==
  Image : Inport
  distance : Inport  Port=2
  Image1 : InportShadow
  ObstacleDetection : Subsystem  Variant=on
  RoadwayDetection : Subsystem  Variant=on
  distance1 : InportShadow  Port=2
  ObstacleAhead : Outport
  AmbientLight : Outport  Port=2
  RoadPathAhead : Outport  Port=3
  wires:
  Image/1 -> ObstacleDetection/1(Image)
  ObstacleDetection/1(ObstacleAhead) -> ObstacleAhead/1
  RoadwayDetection/1(AmbientLight) -> AmbientLight/1
  RoadwayDetection/2(RoadPathAhead) -> RoadPathAhead/1
  distance/1 -> ObstacleDetection/2(distance)
  Image1/1 -> RoadwayDetection/1(Image)
  distance1/1 -> RoadwayDetection/2(distance)

== system Demo002ADAS/RecognitionLayer/VehRecgonition ==
  speed : Inport
  RollYaw : Inport  Port=2
  Mux : Mux  Inputs=2
  VehicleBodyDynamics : Subsystem  Variant=on
  VehicleLongitudinalMotion : Subsystem  Variant=on
  VehMotion : Outport
  wires:
  speed/1 -> VehicleLongitudinalMotion/1(speed_raw)
  RollYaw/1 -> VehicleBodyDynamics/1(RollYaw_raw)
  VehicleBodyDynamics/1(RollYaw) -> Mux/2
  VehicleLongitudinalMotion/1(Speed) -> Mux/1
  Mux/1 -> VehMotion/1

== system Demo002ADAS/Actuators/AHS_Actuator/Actuator_J1 ==
  AHSComannds : Inport
  AHS_Status : Outport

== system Demo002ADAS/Actuators/AHS_Actuator/Actuator_J2 ==
  AHSComannds : Inport
  AHS_Status : Outport

== system Demo002ADAS/Actuators/AHS_Actuator/ToHIL ==
  AHSComannds : Inport
  AHS_Status : Outport

== system Demo002ADAS/Actuators/AHS_Actuator/ToSimulation ==
  AHSComannds : Inport
  AHS_Status_Sim : Inport  Port=2
  AHSCommands_Sim : Outport
  AHS_Status : Outport  Port=2

== system Demo002ADAS/Actuators/Brk_Actuator/Actuator_H1 ==
  BrkComannds : Inport
  Brk_Status : Outport

== system Demo002ADAS/Actuators/Brk_Actuator/Actuator_H2 ==
  BrkComannds : Inport
  Brk_Status : Outport

== system Demo002ADAS/Actuators/Brk_Actuator/ToHIL ==
  BrkComannds : Inport
  Brk_Status : Outport

== system Demo002ADAS/Actuators/Brk_Actuator/ToSimulation ==
  BrkComannds : Inport
  Brk_Status_Sim : Inport  Port=2
  BrkCommands_Sim : Outport
  Brk_Status : Outport  Port=2

== system Demo002ADAS/Actuators/HMI_Device/IP_K1 ==
  HMIComannds : Inport

== system Demo002ADAS/Actuators/HMI_Device/IP_K2 ==
  HMIComannds : Inport

== system Demo002ADAS/Actuators/HMI_Device/ToHIL ==
  HMIComannds : Inport

== system Demo002ADAS/Actuators/HMI_Device/ToSimulation ==
  HMIComannds : Inport
  HMICommands_Sim : Outport

== system Demo002ADAS/Actuators/PT_Actuator/Actuator_G1 ==
  PTComannds : Inport
  PT_Status : Outport

== system Demo002ADAS/Actuators/PT_Actuator/Actuator_G2 ==
  PTComannds : Inport
  PT_Status : Outport

== system Demo002ADAS/Actuators/PT_Actuator/ToHIL ==
  PTComannds : Inport
  PT_Status : Outport

== system Demo002ADAS/Actuators/PT_Actuator/ToSimulation ==
  PTComannds : Inport
  PT_Status_Sim : Inport  Port=2
  PTCommands_Sim : Outport
  PT_Status : Outport  Port=2

== system Demo002ADAS/Actuators/Steering_Actuator/Actuator_I1 ==
  SteeringComannds : Inport
  Steering_Status : Outport

== system Demo002ADAS/Actuators/Steering_Actuator/ToHIL ==
  SteeringComannds : Inport
  Steering_Status : Outport

== system Demo002ADAS/Actuators/Steering_Actuator/ToSimulation ==
  SteeringComannds : Inport
  Steering_Status_Sim : Inport  Port=2
  SteerringCommands_Sim : Outport
  Steering_Status : Outport  Port=2

== system Demo002ADAS/ArbitrationLayer/HMIArbitration/IP_K1 ==
  TrafficSignalAhead : Inport
  HMICommands : Outport

== system Demo002ADAS/ArbitrationLayer/HMIArbitration/IP_K2 ==
  TrafficSignalAhead : Inport
  HMICommands : Outport

== system Demo002ADAS/ArbitrationLayer/HMIArbitration/ToSimulationAndHIL ==
  TrafficSignalAhead : Inport
  HMICommands : Outport

== system Demo002ADAS/ArbitrationLayer/LampLightArbitration/Actuator_J2 ==
  TurnHBOn : Inport
  TurnLBOn : Inport  Port=2
  AdjustHB_LeftRight : Inport  Port=3
  AHSCommands : Outport

== system Demo002ADAS/ArbitrationLayer/LampLightArbitration/ToSimulation, HIL, and Actuator_J1 ==
  TurnHBOn : Inport
  TurnLBOn : Inport  Port=2
  AdjustHB_LeftRight : Inport  Port=3
  AHSCommands : Outport

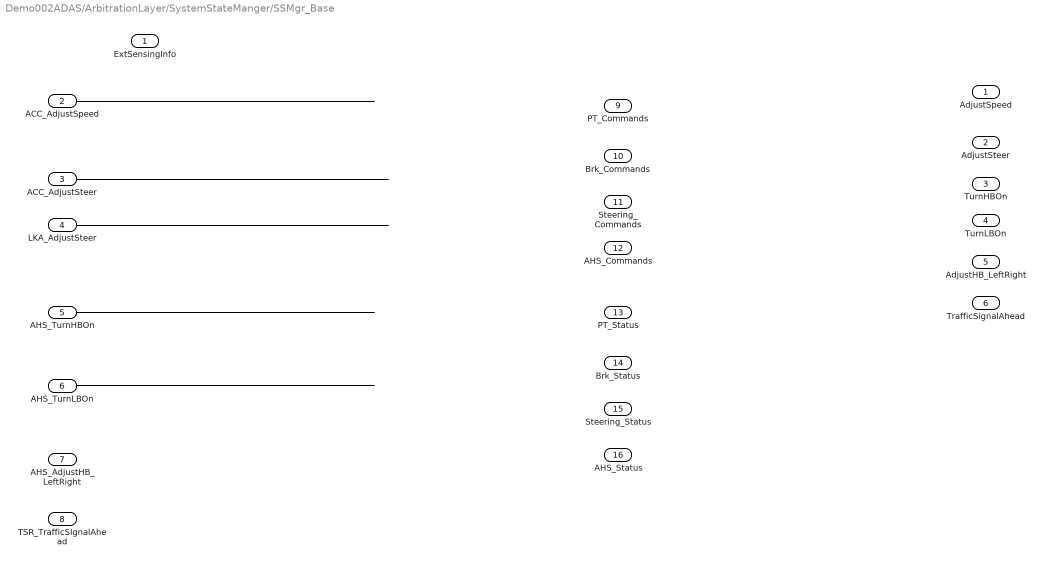
== system Demo002ADAS/ArbitrationLayer/SystemStateManger/SSMgr_Base ==
  ExtSensingInfo : Inport
  ACC_AdjustSpeed : Inport  Port=2
  ACC_AdjustSteer : Inport  Port=3
  LKA_AdjustSteer : Inport  Port=4
  AHS_TurnHBOn : Inport  Port=5
  AHS_TurnLBOn : Inport  Port=6
  AHS_AdjustHB_LeftRight : Inport  Port=7
  TSR_TrafficSIgnalAhead : Inport  Port=8
  PT_Commands : Inport  Port=9
  Brk_Commands : Inport  Port=10
  Steering_Commands : Inport  Port=11
  AHS_Commands : Inport  Port=12
  PT_Status : Inport  Port=13
  Brk_Status : Inport  Port=14
  Steering_Status : Inport  Port=15
  AHS_Status : Inport  Port=16
  AdjustSpeed : Outport
  AdjustSteer : Outport  Port=2
  TurnHBOn : Outport  Port=3
  TurnLBOn : Outport  Port=4
  AdjustHB_LeftRight : Outport  Port=5
  TrafficSignalAhead : Outport  Port=6
  wires:
  AHS_TurnHBOn/1 -> ?
  ACC_AdjustSpeed/1 -> ?
  AHS_TurnLBOn/1 -> ?
  ACC_AdjustSteer/1 -> ?
  LKA_AdjustSteer/1 -> ?

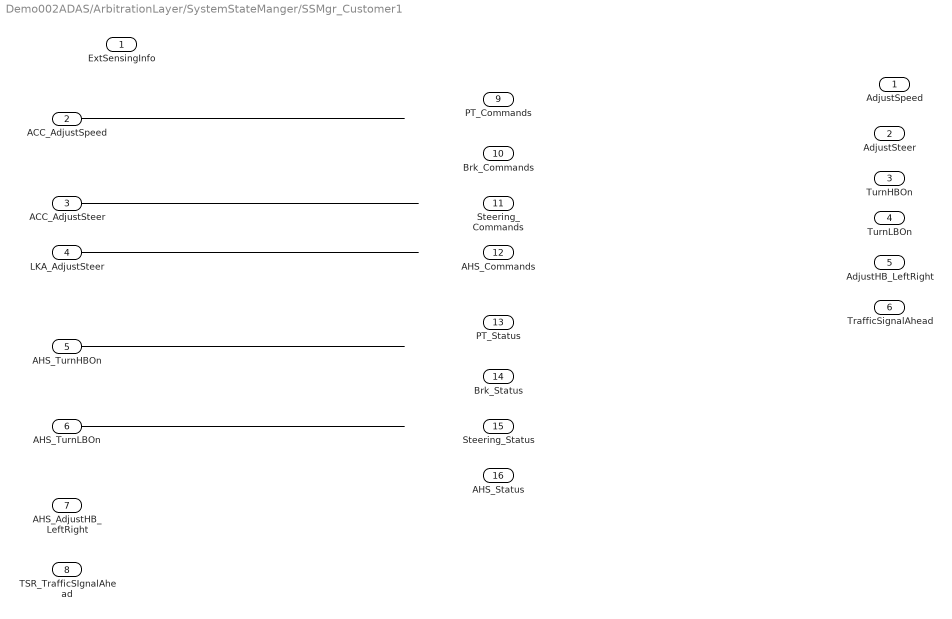
== system Demo002ADAS/ArbitrationLayer/SystemStateManger/SSMgr_Customer1 ==
  ExtSensingInfo : Inport
  ACC_AdjustSpeed : Inport  Port=2
  ACC_AdjustSteer : Inport  Port=3
  LKA_AdjustSteer : Inport  Port=4
  AHS_TurnHBOn : Inport  Port=5
  AHS_TurnLBOn : Inport  Port=6
  AHS_AdjustHB_LeftRight : Inport  Port=7
  TSR_TrafficSIgnalAhead : Inport  Port=8
  PT_Commands : Inport  Port=9
  Brk_Commands : Inport  Port=10
  Steering_Commands : Inport  Port=11
  AHS_Commands : Inport  Port=12
  PT_Status : Inport  Port=13
  Brk_Status : Inport  Port=14
  Steering_Status : Inport  Port=15
  AHS_Status : Inport  Port=16
  AdjustSpeed : Outport
  AdjustSteer : Outport  Port=2
  TurnHBOn : Outport  Port=3
  TurnLBOn : Outport  Port=4
  AdjustHB_LeftRight : Outport  Port=5
  TrafficSignalAhead : Outport  Port=6
  wires:
  LKA_AdjustSteer/1 -> ?
  ACC_AdjustSteer/1 -> ?
  AHS_TurnLBOn/1 -> ?
  ACC_AdjustSpeed/1 -> ?
  AHS_TurnHBOn/1 -> ?

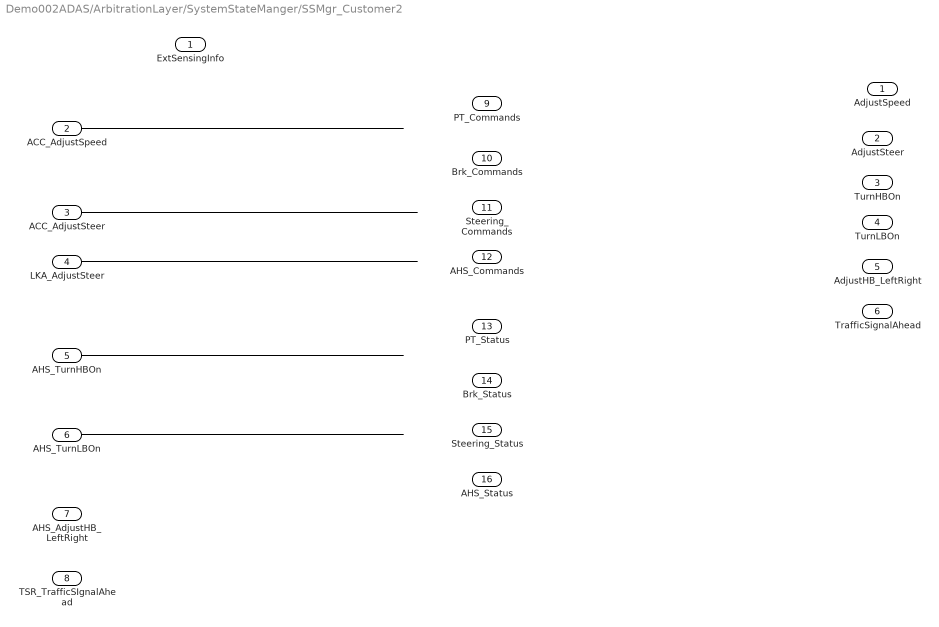
== system Demo002ADAS/ArbitrationLayer/SystemStateManger/SSMgr_Customer2 ==
  ExtSensingInfo : Inport
  ACC_AdjustSpeed : Inport  Port=2
  ACC_AdjustSteer : Inport  Port=3
  LKA_AdjustSteer : Inport  Port=4
  AHS_TurnHBOn : Inport  Port=5
  AHS_TurnLBOn : Inport  Port=6
  AHS_AdjustHB_LeftRight : Inport  Port=7
  TSR_TrafficSIgnalAhead : Inport  Port=8
  PT_Commands : Inport  Port=9
  Brk_Commands : Inport  Port=10
  Steering_Commands : Inport  Port=11
  AHS_Commands : Inport  Port=12
  PT_Status : Inport  Port=13
  Brk_Status : Inport  Port=14
  Steering_Status : Inport  Port=15
  AHS_Status : Inport  Port=16
  AdjustSpeed : Outport
  AdjustSteer : Outport  Port=2
  TurnHBOn : Outport  Port=3
  TurnLBOn : Outport  Port=4
  AdjustHB_LeftRight : Outport  Port=5
  TrafficSignalAhead : Outport  Port=6
  wires:
  AHS_TurnHBOn/1 -> ?
  ACC_AdjustSpeed/1 -> ?
  AHS_TurnLBOn/1 -> ?
  ACC_AdjustSteer/1 -> ?
  LKA_AdjustSteer/1 -> ?

== system Demo002ADAS/ArbitrationLayer/VehicleMotionControl/ForeAftMotion ==
  note: 1) Only subsystems can be added as variant choices at this level
      | 2) Blocks cannot be connected at this level as connectivity is
      | automatically determined at simulation, based on the active variant
  AdjustSpeed : Inport
  VehForeAft_G2,H2 : Subsystem  VariantControl=D2_AL_VMC_FAM_VehForeAft_G2_H2
  "VehForeAft_Simulation, HIL, Actuators G1,H1 and G1,H2" : Subsystem  VariantControl=D2_AL_VMC_FAM_VehForeAft_Simulation_HIL_Act_G1_H1_and_G1_H2
  PTCommands : Outport
  BrkCommands : Outport  Port=2

== system Demo002ADAS/ArbitrationLayer/VehicleMotionControl/LeftRightMotion ==
  note: 1) Only subsystems can be added as variant choices at this level
      | 2) Blocks cannot be connected at this level as connectivity is
      | automatically determined at simulation, based on the active variant
  AdjustSteer : Inport
  Actuator_I1 : Subsystem  VariantControl=D2_AL_VMC_LRM_Actuator_J1
  SimulationAndHIL : Subsystem  VariantControl=D2_AL_VMC_LRM_SimulationAndHIL
  SteeringCommands : Outport

== system Demo002ADAS/ExternalSensing/Camera/FromHIL ==
  Image : Outport

== system Demo002ADAS/ExternalSensing/Camera/FromSimulation ==
  ImageSim : Inport
  Image : Outport
  wires:
  ImageSim/1 -> Image/1

== system Demo002ADAS/ExternalSensing/Camera/Sensor_C1 ==
  Image : Outport

== system Demo002ADAS/ExternalSensing/Camera/Sensor_C2 ==
  Image : Outport

== system Demo002ADAS/ExternalSensing/Lidar/FromHIL ==
  Lidar : Outport

== system Demo002ADAS/ExternalSensing/Lidar/FromSimulation ==
  LidarSim : Inport
  Lidar : Outport
  wires:
  LidarSim/1 -> Lidar/1

== system Demo002ADAS/ExternalSensing/Lidar/Sensor_B1 ==
  Lidar : Outport

== system Demo002ADAS/ExternalSensing/Lidar/Sensor_B2 ==
  Lidar : Outport

== system Demo002ADAS/ExternalSensing/mmWaveRadar/FromHIL ==
  mmWv : Outport

== system Demo002ADAS/ExternalSensing/mmWaveRadar/FromSimulation ==
  mmWvSim : Inport
  mmWv : Outport
  wires:
  mmWvSim/1 -> mmWv/1

== system Demo002ADAS/ExternalSensing/mmWaveRadar/Sensor_A1 ==
  mmWv : Outport

== system Demo002ADAS/ExternalSensing/mmWaveRadar/Sensor_A2 ==
  mmWv : Outport

== system Demo002ADAS/InternalSensing/GPS/FromHIL ==
  Speed : Outport

== system Demo002ADAS/InternalSensing/GPS/FromSimulation ==
  SpeedSim : Inport
  Speed : Outport
  wires:
  SpeedSim/1 -> Speed/1

== system Demo002ADAS/InternalSensing/GPS/GPS_E1 ==
  Speed : Outport

== system Demo002ADAS/InternalSensing/GPS/GPS_E2 ==
  Speed : Outport

== system Demo002ADAS/InternalSensing/RollYawSensing/FromHIL ==
  RollYaw : Outport

== system Demo002ADAS/InternalSensing/RollYawSensing/FromSimulation ==
  RollYawSim : Inport
  RollYaw : Outport
  wires:
  RollYawSim/1 -> RollYaw/1

== system Demo002ADAS/InternalSensing/RollYawSensing/Sensor_F1 ==
  RollYaw : Outport

== system Demo002ADAS/InternalSensing/VehicleSpeedSensing/FromComm ==
  Speed : Outport

== system Demo002ADAS/InternalSensing/VehicleSpeedSensing/FromHIL ==
  Speed : Outport

== system Demo002ADAS/InternalSensing/VehicleSpeedSensing/FromSimulation ==
  SpeedSim : Inport
  Speed : Outport
  wires:
  SpeedSim/1 -> Speed/1

== system Demo002ADAS/InternalSensing/VehicleSpeedSensing/Sensor_D1 ==
  Speed : Outport

== system Demo002ADAS/InternalSensing/VehicleSpeedSensing/Sensor_D2 ==
  Speed : Outport

== system Demo002ADAS/MajorFunctionsLayer/ACC/ACC_Complex ==
  ObstacleAhead : Inport
  VehMotion : Inport  Port=2
  RoadPathAhead : Inport  Port=3
  AdjustSpeed : Outport
  AdjustSteer : Outport  Port=2
  wires:
  ObstacleAhead/1 -> AdjustSpeed/1

== system Demo002ADAS/MajorFunctionsLayer/ACC/ACC_Simple ==
  ObstacleAhead : Inport
  VehMotion : Inport  Port=2
  AdjustSpeed : Outport
  wires:
  ObstacleAhead/1 -> AdjustSpeed/1

== system Demo002ADAS/MajorFunctionsLayer/AHS/AHB_advanced ==
  AmbientLight : Inport
  TurnHBOn : Outport
  TurnLBOn : Outport  Port=2
  wires:
  AmbientLight/1 -> TurnHBOn/1

== system Demo002ADAS/MajorFunctionsLayer/AHS/AHB_simple ==
  AmbientLight : Inport
  TurnHLOn : Outport
  wires:
  AmbientLight/1 -> TurnHLOn/1

== system Demo002ADAS/MajorFunctionsLayer/AHS/AHS ==
  AmbientLight : Inport
  RoadPathAhead : Inport  Port=2
  TurnHBOn : Outport
  TurnLBOn : Outport  Port=2
  AdjustHB_LeftRight : Outport  Port=3
  wires:
  AmbientLight/1 -> TurnHBOn/1

== system Demo002ADAS/MajorFunctionsLayer/LKA/LKA ==
  VehMotion : Inport
  RoadPathAhead : Inport  Port=2
  AdjustSteer : Outport

== system Demo002ADAS/MajorFunctionsLayer/TSR/TSR_Germany ==
  ObstacleAhead : Inport
  TrafficSignAhead : Outport

== system Demo002ADAS/MajorFunctionsLayer/TSR/TSR_Japan ==
  ObstacleAhead : Inport
  TrafficSignAhead : Outport

== system Demo002ADAS/MajorFunctionsLayer/TSR/TSR_UK ==
  ObstacleAhead : Inport
  TrafficSignAhead : Outport

== system Demo002ADAS/MajorFunctionsLayer/TSR/TSR_US ==
  ObstacleAhead : Inport
  TrafficSignAhead : Outport

== system Demo002ADAS/RecognitionLayer/EnvRecognition/ObstacleDetection ==
  note: 1) Only subsystems can be added as variant choices at this level
      | 2) Blocks cannot be connected at this level as connectivity is
      | automatically determined at simulation, based on the active variant
  Image : Inport
  distance : Inport  Port=2
  LidarSystemNoCamera : Subsystem  VariantControl=D2_RL_EnvRec_ObsDet_LidarSystemNoCamera
  LidarSystemPlusCamera : Subsystem  VariantControl=D2_RL_EnvRec_ObsDet_LidarSystemPlusCamera
  mmWvSystemNoCamera : Subsystem  VariantControl=D2_RL_EnvRec_ObsDet_mmWvSystemNoCamera
  mmWvSystemPlusCamera : Subsystem  VariantControl=D2_RL_EnvRec_ObsDet_mmWvSystemPlusCamera
  mmWwAndLidarNoCamera : Subsystem  VariantControl=D2_RL_EnvRec_ObsDet_mmWwAndLidarNoCamera
  mmWwAndLidarPlusCamera : Subsystem  VariantControl=D2_RL_EnvRec_ObsDet_mmWwAndLidarPlusCamera
  ObstacleAhead : Outport

== system Demo002ADAS/RecognitionLayer/EnvRecognition/RoadwayDetection ==
  note: 1) Only subsystems can be added as variant choices at this level
      | 2) Blocks cannot be connected at this level as connectivity is
      | automatically determined at simulation, based on the active variant
  Image : Inport
  distance : Inport  Port=2
  CameraOnly : Subsystem  VariantControl=D2_RL_EnvRec_RoadDet_CameraOnly
  CameraPlusLidarSystem : Subsystem  VariantControl=D2_RL_EnvRec_RoadDet_CameraPlusLidarSystem
  CameraPlusLidarSystemAndmWvSystem : Subsystem  VariantControl=D2_RL_EnvRec_RoadDet_CameraPlusLidarSystemAndmWvSystem
  CameraPlusmmWvSystem : Subsystem  VariantControl=D2_RL_EnvRec_RoadDet_CameraPlusmmWvSystem
  AmbientLight : Outport
  RoadPathAhead : Outport  Port=2

== system Demo002ADAS/RecognitionLayer/VehRecgonition/VehicleBodyDynamics ==
  note: 1) Only subsystems can be added as variant choices at this level
      | 2) Blocks cannot be connected at this level as connectivity is
      | automatically determined at simulation, based on the active variant
  RollYaw_raw : Inport
  BaseFiltersForF1 : Subsystem  VariantControl=D2_RL_VehRec_VBD_BaseFiltersForF1
  BaseFiltersForSimulationAndHIL : Subsystem  VariantControl=D2_RL_VehRec_VBD_BaseFiltersForSimulationAndHIL
  RollYaw : Outport

== system Demo002ADAS/RecognitionLayer/VehRecgonition/VehicleLongitudinalMotion ==
  note: 1) Only subsystems can be added as variant choices at this level
      | 2) Blocks cannot be connected at this level as connectivity is
      | automatically determined at simulation, based on the active variant
  speed_raw : Inport
  GPSOnly : Subsystem  VariantControl=D2_RL_VehRec_VLM_GPSOnly
  SensedAndGPS : Subsystem  VariantControl=D2_RL_VehRec_VLM_SensedAndGPS
  SensedOnly : Subsystem  VariantControl=D2_RL_VehRec_VLM_SensedOnly
  Speed : Outport

== system Demo002ADAS/ArbitrationLayer/VehicleMotionControl/ForeAftMotion/VehForeAft_G2,H2 ==
  AdjustSpeed : Inport
  PTCommands : Outport
  BrkCommands : Outport  Port=2

== system Demo002ADAS/ArbitrationLayer/VehicleMotionControl/ForeAftMotion/VehForeAft_Simulation, HIL, Actuators G1,H1 and G1,H2 ==
  AdjustSpeed : Inport
  PTCommands : Outport
  BrkCommands : Outport  Port=2

== system Demo002ADAS/ArbitrationLayer/VehicleMotionControl/LeftRightMotion/Actuator_I1 ==
  AdjustSteer : Inport
  SteeringCommands : Outport

== system Demo002ADAS/ArbitrationLayer/VehicleMotionControl/LeftRightMotion/SimulationAndHIL ==
  AdjustSteer : Inport
  SteeringCommands : Outport

== system Demo002ADAS/RecognitionLayer/EnvRecognition/ObstacleDetection/LidarSystemNoCamera ==
  distance : Inport
  ObstacleAhead : Outport

== system Demo002ADAS/RecognitionLayer/EnvRecognition/ObstacleDetection/LidarSystemPlusCamera ==
  Image : Inport
  distance : Inport  Port=2
  ObstacleAhead : Outport

== system Demo002ADAS/RecognitionLayer/EnvRecognition/ObstacleDetection/mmWvSystemNoCamera ==
  distance : Inport
  ObstacleAhead : Outport

== system Demo002ADAS/RecognitionLayer/EnvRecognition/ObstacleDetection/mmWvSystemPlusCamera ==
  Image : Inport
  distance : Inport  Port=2
  ObstacleAhead : Outport

== system Demo002ADAS/RecognitionLayer/EnvRecognition/ObstacleDetection/mmWwAndLidarNoCamera ==
  distance : Inport
  ObstacleAhead : Outport

== system Demo002ADAS/RecognitionLayer/EnvRecognition/ObstacleDetection/mmWwAndLidarPlusCamera ==
  Image : Inport
  distance : Inport  Port=2
  ObstacleAhead : Outport

== system Demo002ADAS/RecognitionLayer/EnvRecognition/RoadwayDetection/CameraOnly ==
  Image : Inport
  AmbientLight : Outport
  RoadPathAhead : Outport  Port=2

== system Demo002ADAS/RecognitionLayer/EnvRecognition/RoadwayDetection/CameraPlusLidarSystem ==
  Image : Inport
  distance : Inport  Port=2
  AmbientLight : Outport
  RoadPathAhead : Outport  Port=2

== system Demo002ADAS/RecognitionLayer/EnvRecognition/RoadwayDetection/CameraPlusLidarSystemAndmWvSystem ==
  Image : Inport
  distance : Inport  Port=2
  AmbientLight : Outport
  RoadPathAhead : Outport  Port=2

== system Demo002ADAS/RecognitionLayer/EnvRecognition/RoadwayDetection/CameraPlusmmWvSystem ==
  Image : Inport
  distance : Inport  Port=2
  AmbientLight : Outport
  RoadPathAhead : Outport  Port=2

== system Demo002ADAS/RecognitionLayer/VehRecgonition/VehicleBodyDynamics/BaseFiltersForF1 ==
  RollYaw_raw : Inport
  RollYaw : Outport

== system Demo002ADAS/RecognitionLayer/VehRecgonition/VehicleBodyDynamics/BaseFiltersForSimulationAndHIL ==
  RollYaw_raw : Inport
  RollYaw : Outport

== system Demo002ADAS/RecognitionLayer/VehRecgonition/VehicleLongitudinalMotion/GPSOnly ==
  speed_raw : Inport
  Speed : Outport

== system Demo002ADAS/RecognitionLayer/VehRecgonition/VehicleLongitudinalMotion/SensedAndGPS ==
  speed_raw : Inport
  Speed : Outport

== system Demo002ADAS/RecognitionLayer/VehRecgonition/VehicleLongitudinalMotion/SensedOnly ==
  speed_raw : Inport
  Speed : Outport
